simulink model "SpeedSimulationHW"  (R2013b)
settings: Solver=FixedStepDiscrete  SolverMode=SingleTasking  StartTime=0.0  StopTime=3000  FixedStep=0.1  RelTol=1e-3
undefined symbols (not defined in the file or in its folder): Sensor, spartan500lap_lib
libraries: xbsIndex_r4 x42, simulink x3
settings Model: Creator=laca  LastModifiedBy=laca

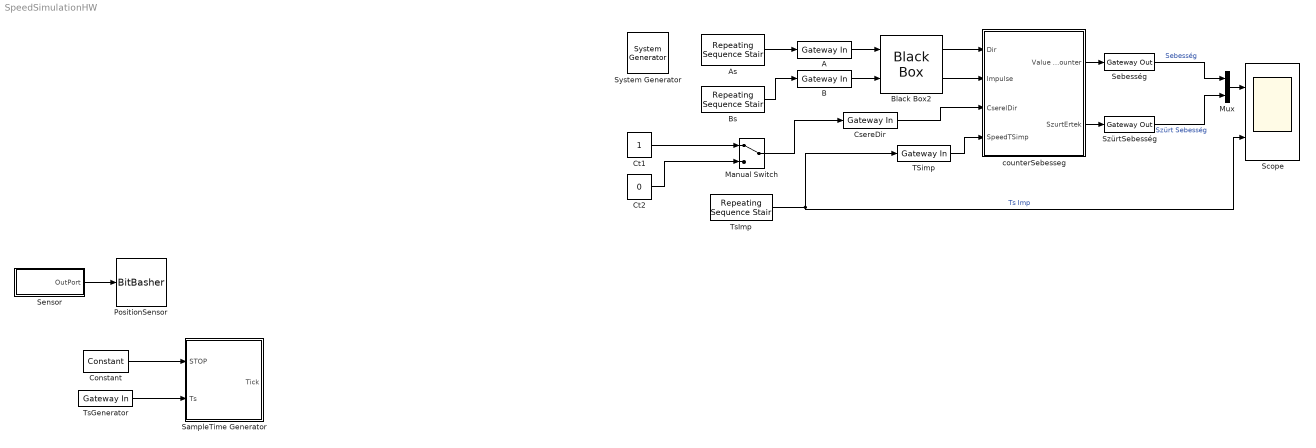
== system SpeedSimulationHW ==
  " System Generator" : xbsIndex_r4/ System Generator  Tag=genX  xilinxfamily=spartan3e  part=xc3s500e  speed=-4  package=pq208  synthesis_tool=XST  clock_wrapper=Clock Enables  directory=./netlist  proj_type=Project Navigator  Synth_file=XST Defaults  Impl_file=ISE Defaults  testbench=off  simulink_period=1  sysclk_period=20  dcm_input_clock_period=10  incr_netlist=off  trim_vbits=Everywhere in SubSystem  dbl_ovrd=According to Block Masks  core_generation=According to Block Masks  run_coregen=off  deprecated_control=off  eval_field=0  block_type=sysgen
  A : xbsIndex_r4/Gateway In  gui_display_data_type=Boolean  arith_type=Boolean  n_bits=16  bin_pt=14  preci_type=Single  exp_width=8  frac_width=24  quantization="Round  (unbiased: +/- Inf)"  overflow=Saturate  period=1  dbl_ovrd=off  timing_constraint=None  locs_specified=off  LOCs={}  UseAsADC=off  ADCChannel='1'  inherit_from_input=off  hdl_port=on  block_type=gatewayin
  As : simulink/Sources/Repeating Sequence Stair  OutValues="[ 0 0 1 1 1 1 1 0 0 0  0 0 1 1 1 1 1 0 0 0  0 0 1 1 1 1 1 0 0 0  0 0 1 1 1 1 1 0 0 0  0 0 1 1 1 1 1 0 0 0  0 0 1 1 1 1 1 0 0 0  0 0 1 1 1 1 1 0 0 0  0 0 1 1 1 1 1 0 0 0  0 0 1 1 1 1 1 0 0 0  0 0 1 1 1 1 1 0 0 0  0 0 1 1 1 1 1 0 0 0 0 0 1 1 1 1 1 0 0 0 0 0 1 1 1 1 1 0 0 0 0 0 1 1 1 1 1 0 0 0 1 1 1 1 1 0 0 0 0 0 1 1 1 1 1 0 0 0 0 0 1 1 1 1 1 0 0 0 0 0 1 1 1 1 1 0 0 0 0 0 0 0 0 1 1  0 0 0 0 0 0 0 0 1 1 0 0 0 0 0 0 0 0 1 1  0 0 0 0 0 0 0 0 1 1 0 0 0 0 0 0 0 0 0 0 0 0 0 0 0 0 0 0 0 0 0 0 0 0 0 0 0 0 0 0 0 0 0 0 0 0 0 0 0 0 0 0 0 0 0 0 1 1 0 0 0 0 0 0 0 0 1 1 0 0 0 0 0 0 0 0 1 1 0 0 0 0 ].'"  tsamp=1  OutMin=[]  OutMax=[]  OutDataTypeStr=double  OutputDataTypeScalingMode=double  OutDataType=fixdt(0,8)  ConRadixGroup=Best Precision: Vector-wise  OutScaling=2^-12
  B : xbsIndex_r4/Gateway In  gui_display_data_type=Boolean  arith_type=Boolean  n_bits=16  bin_pt=14  preci_type=Single  exp_width=8  frac_width=24  quantization="Round  (unbiased: +/- Inf)"  overflow=Saturate  period=1  dbl_ovrd=off  timing_constraint=None  locs_specified=off  LOCs={}  UseAsADC=off  ADCChannel='1'  inherit_from_input=off  hdl_port=on  block_type=gatewayin
  Black Box2 : xbsIndex_r4/Black Box  init_code=IncSensor_config  sim_method=ISE Simulator  verbose=off  block_type=blackbox2
  Bs : simulink/Sources/Repeating Sequence Stair  OutValues="[1 1 1 1 1 0 0 0 0 0 1 1 1 1 1 0 0 0 0 0 1 1 1 1 1 0 0 0 0 0 1 1 1 1 1 0 0 0 0 0 1 1 1 1 1 0 0 0 0 0 1 1 1 1 1 0 0 0 0 0 1 1 1 1 1 0 0 0 0 0 1 1 1 1 1 0 0 0 0 0 1 1 1 1 1 0 0 0 0 0 1 1 1 1 1 0 0 0 0 0 1 1 1 1 1 0 0 0 0 0 1 1 1 1 1 0 0 0 0 0 1 1 1 1 1 0 0 0 0 0 1 1 1 1 1 0 0 0 0 0 0 1 1 1 1 1 0 0 0 0 0 1 1 1 1 1 0 0 0 0 0 1 1 1 1 1 0 0 0 0 0 1 1 1 1 1 0 0 0  0 0 1 1 1 1 1 0 0 0  0 0 1 1 1 1 1 0 0 0  0 0 1 1 1 1 1 0 0 0  0 0 1 1 1 1 1 0 0 0  0 0 1 1 1 1 1 0 0 0  0 0 1 1 1 1 1 0 0 0 0 0 0 0 0 0 0 0 0 0 0 0 0 0 0 1 1 1 1 1 1 1 1 1 1 1 1 1 1 1 1 1 1 1 1 1 1 1 1 1 1 1 1 1 1].'"  tsamp=1  OutMin=[]  OutMax=[]  OutDataTypeStr=double  OutputDataTypeScalingMode=double  OutDataType=fixdt(0,8)  ConRadixGroup=Best Precision: Vector-wise  OutScaling=2^-12
  Constant : xbsIndex_r4/Constant  const=0  gui_display_data_type=Boolean  arith_type=Boolean  n_bits=16  bin_pt=14  preci_type=Single  exp_width=8  frac_width=24  explicit_period=off  period=1  equ=P=C  opselect=C  inp2=PCIN>>17  opr=+  inp1=P  carry=CIN  dbl_ovrd=off  block_type=constant
  CsereDir : xbsIndex_r4/Gateway In  gui_display_data_type=Boolean  arith_type=Boolean  n_bits=16  bin_pt=14  preci_type=Single  exp_width=8  frac_width=24  quantization="Round  (unbiased: +/- Inf)"  overflow=Saturate  period=1  dbl_ovrd=off  timing_constraint=None  locs_specified=off  LOCs={}  UseAsADC=off  ADCChannel='1'  inherit_from_input=off  hdl_port=on  block_type=gatewayin
  Ct1 : Constant
  Ct2 : Constant  Value=0
  Manual Switch : ManualSwitch
  Mux : Mux  Inputs=2
  PositionSensor : xbsIndex_r4/BitBasher  bitexpr=|  display_expr=off  sr_1=1  arith_type1=Unsigned  bin_pt1=0  sr_2=2  arith_type2=Unsigned  bin_pt2=0  sr_3=3  arith_type3=Unsigned  bin_pt3=0  sr_4=4  arith_type4=Unsigned  bin_pt4=0  dbl_ovrd=off  block_type=bitbasher
      | <!DOCTYPE HTML PUBLIC "-//W3C//DTD HTML 4.0//EN" "http://www.w3.org/TR/REC-html40/strict.dtd">
      | <html><head><meta name="qrichtext" content="1" /><style type="text/css">
      | p, li { white-space: pre-wrap; }
      | </style></head><body style=" font-family:'MS Shell Dlg 2'; font-size:8.25pt; font-weight:400; font-style:normal;">
      | <p style=" margin-top:12px; margin-bottom:12px; margin-left:0px; margin-right:0px; -qt-block-indent:0; text-indent:0px;"><span style=" font-family:'MS Shell Dlg'; font-size:8pt;">A={a[2]}<br />B={a[3]}</span></p></body></html>
  SampleTime Generator : Subsystem
  Scope : Scope  NumInputPorts=2
      settings: TickLabels=on  ShowLegends=on  YMin=225.15~-1  YMax=248.85~1
  Sebesség : xbsIndex_r4/Gateway Out  inherit_from_input=off  hdl_port=on  timing_constraint=None  locs_specified=off  LOCs={}  UseAsDAC=off  DACChannel='1'  block_type=gatewayout
  Sensor : Subsystem  AncestorBlock=spartan500lap_lib/Sensor  mask(Non-Memory-Mapped Input Port){signed=off, bpt=0, show_in=off, c=0}
      mask prompts: signed "Signed  (2's comp)"; bpt "Binary Point"; show_in "Provide Input Double"; c "Constant for Simulation"
      mask help:
      | Port Name: "Sensor"
      | Port Type: 5-bit Vector
      mask init:
      | [bg,fg] = xlcmap('IO',0);
      | iPos = get_param(gcb,'Position');
      | iWidth=iPos(3)-iPos(1);
      | iHeight=iPos(4)-iPos(2);
      | [logoX, logoY] = xlogo(iPos);
      | if (signed)
      |     set_param([gcb '/Sensor'],'arith_type','Signed  (2''s comp)');
      | else
      |     set_param([gcb '/Sensor'],'arith_type','Unsigned');
      | end
      | if (show_in)
      |     old = find_system(gcb, 'LookUnderMasks', 'all', 'Name', 'Constant');
      |     if (length(old) > 0)
      |         replace_block(gcb, 'Name', 'Constant', 'InPort', 'noprompt');
      |         set_param([gcb '/Constant'], 'Name', 'InPort');
      |     end
      |     portdir = 'input';
      |     portstr = 'dbl';
      | else
      |     old = find_system(gcb, 'LookUnderMasks', 'all', 'Name', 'InPort');
      |     if (length(old) > 0)
      |         replace_block(gcb, 'Name', 'InPort', 'Constant', 'noprompt');
      |         set_param([gcb '/InPort'], 'Name', 'Constant');
      |         set_param([gcb '/Constant'], 'Value', 'c');
      |     end
      |     portdir = 'output';
      |     portstr = '';
      | end
      settings: CopyFcn=set_param(gcb,'LinkStatus','inactive');
      mask Callback show_in:
      | mask_vis = get_param(gcb, 'MaskVisibilities');
      | if (strcmp(get_param(gcb, 'show_in'),'on'))
      |     mask_vis(4) = {'off'};
      | else
      |     mask_vis(4) = {'on'};
      | end
      | set_param(gcb, 'MaskVisibilities', mask_vis);
      mask Display:
      | patch([0 iWidth iWidth 0],[0 0 iHeight iHeight] , bg);
      | patch(logoX,logoY, fg);
      | plot([0 0 iWidth iWidth 0], [0 iHeight iHeight 0 0]);
      | port_label(portdir,1,portstr);
      | port_label('output',1,'Sensor');
      | text(2,5,'nmm');
  SzürtSebesség : xbsIndex_r4/Gateway Out  inherit_from_input=off  hdl_port=on  timing_constraint=None  locs_specified=off  LOCs={}  UseAsDAC=off  DACChannel='1'  block_type=gatewayout
  TSimp : xbsIndex_r4/Gateway In  gui_display_data_type=Boolean  arith_type=Boolean  n_bits=16  bin_pt=14  preci_type=Single  exp_width=8  frac_width=24  quantization="Round  (unbiased: +/- Inf)"  overflow=Saturate  period=1  dbl_ovrd=off  timing_constraint=None  locs_specified=off  LOCs={}  UseAsADC=off  ADCChannel='1'  inherit_from_input=off  hdl_port=on  block_type=gatewayin
  TsGenerator : xbsIndex_r4/Gateway In  gui_display_data_type=Fixed-point  arith_type="Signed  (2's comp)"  n_bits=16  bin_pt=14  preci_type=Single  exp_width=8  frac_width=24  quantization="Round  (unbiased: +/- Inf)"  overflow=Saturate  period=1  dbl_ovrd=off  timing_constraint=None  locs_specified=off  LOCs={}  UseAsADC=off  ADCChannel='1'  inherit_from_input=off  hdl_port=on  block_type=gatewayin
  TsImp : simulink/Sources/Repeating Sequence Stair  OutValues=[zeros(1,50) 1 ].'  tsamp=1  OutMin=[]  OutMax=[]  OutDataTypeStr=double  OutputDataTypeScalingMode=double  OutDataType=fixdt(0,8)  ConRadixGroup=Best Precision: Vector-wise  OutScaling=2^-12
  counterSebesseg : Subsystem
  wires:
  Sensor/1(OutPort) -> PositionSensor/1
  Constant/1 -> SampleTime Generator/1(STOP)
  TsGenerator/1 -> SampleTime Generator/2(Ts)
  Bs/1 -> B/1
  As/1 -> A/1
  A/1 -> Black Box2/1
  B/1 -> Black Box2/2
  Black Box2/1 -> counterSebesseg/1(Dir)
  Black Box2/2 -> counterSebesseg/2(Impulse)
  TSimp/1 -> counterSebesseg/4(SpeedTSimp)
  CsereDir/1 -> counterSebesseg/3(CserelDir)
  counterSebesseg/2(SzurtErtek) -> SzürtSebesség/1
  TsImp/1 -> TSimp/1, Scope/2  "Ts Imp"
  Ct1/1 -> Manual Switch/1
  Ct2/1 -> Manual Switch/2
  Sebesség/1 -> Mux/1  "Sebesség"
  SzürtSebesség/1 -> Mux/2  "Szürt Sebesség"
  Mux/1 -> Scope/1
  Manual Switch/1 -> CsereDir/1
  counterSebesseg/1(Value Counter) -> Sebesség/1

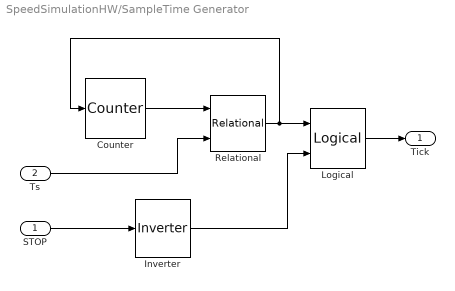
== system SpeedSimulationHW/SampleTime Generator ==
  STOP : Inport
  Ts : Inport  Port=2
  Counter : xbsIndex_r4/Counter  cnt_type=Free Running  cnt_to=Inf  operation=Up  start_count=0  cnt_by_val=1  arith_type=Unsigned  n_bits=32  bin_pt=0  load_pin=off  rst=on  en=off  explicit_period=on  period=1  dbl_ovrd=off  use_behavioral_HDL=off  implementation=Fabric  block_type=counter
  Inverter : xbsIndex_r4/Inverter  en=off  latency=0  dbl_ovrd=off  block_type=inv
  Logical : xbsIndex_r4/Logical  logical_function=AND  inputs=2  en=off  latency=0  precision=Full  arith_type=Unsigned  n_bits=16  bin_pt=0  align_bp=on  dbl_ovrd=off  block_type=logical
  Relational : xbsIndex_r4/Relational  mode=a=b  en=off  latency=0  dbl_ovrd=off  block_type=relational
  Tick : Outport
  wires:
  Ts/1 -> Relational/2
  Counter/1 -> Relational/1
  Relational/1 -> Logical/1, Counter/1
  Logical/1 -> Tick/1
  STOP/1 -> Inverter/1
  Inverter/1 -> Logical/2

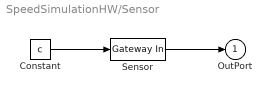
== system SpeedSimulationHW/Sensor ==
  Constant : Constant  Value=c
  Sensor : xbsIndex_r4/Gateway In  gui_display_data_type=Fixed-point  arith_type=Unsigned  n_bits=5  bin_pt=max(0,min(bpt,5))  preci_type=Single  exp_width=8  frac_width=24  quantization="Round  (unbiased: +/- Inf)"  overflow=Saturate  period=1  dbl_ovrd=off  timing_constraint=None  locs_specified=on  LOCs={'P112','P113','P115','P116','P119'}  UseAsADC=off  ADCChannel='1'  inherit_from_input=off  hdl_port=on  block_type=gatewayin
      settings: sginterface={'Xilinx'=>{'jtaghwcosim'=>{'non_memory_mapped_port'=>'Sensor'}}}
  OutPort : Outport
  wires:
  Sensor/1 -> OutPort/1
  Constant/1 -> Sensor/1

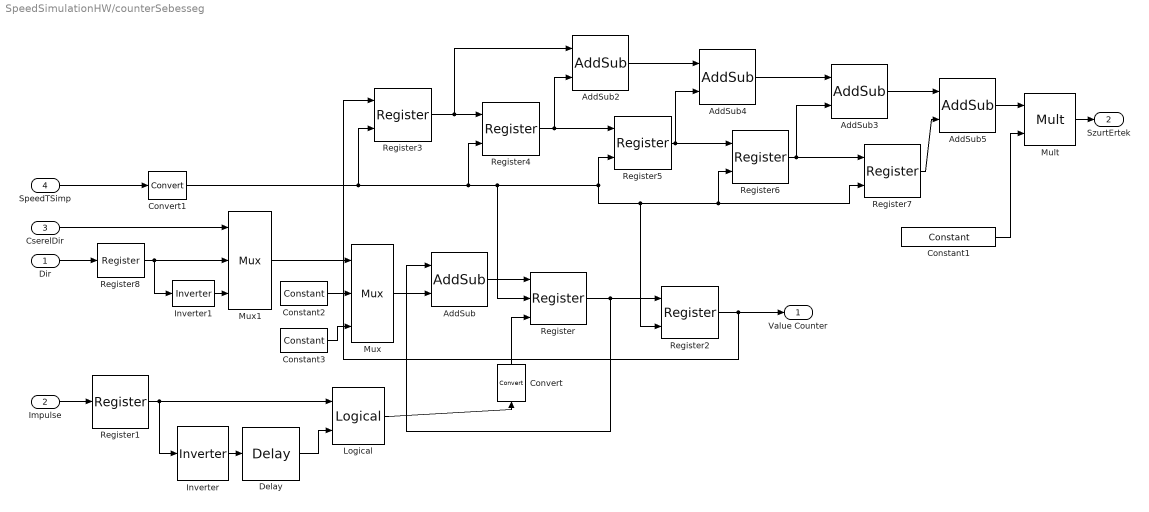
== system SpeedSimulationHW/counterSebesseg ==
  Dir : Inport
  Impulse : Inport  Port=2
  CserelDir : Inport  Port=3
  SpeedTSimp : Inport  Port=4
  AddSub{,2..5} (5 alike) : xbsIndex_r4/AddSub  mode=Addition  use_carryin=off  use_carryout=off  en=off  latency=0  precision=User Defined  arith_type="Signed  (2's comp)"  n_bits=16  bin_pt=0  quantization=Truncate  overflow=Saturate  dbl_ovrd=off  use_behavioral_HDL=off  hw_selection=Fabric  pipelined=off  block_type=addsub
  Constant1 : xbsIndex_r4/Constant  const=1/5  gui_display_data_type=Fixed-point  arith_type=Signed (2's comp)  n_bits=16  bin_pt=14  preci_type=Single  exp_width=8  frac_width=24  explicit_period=off  period=1  equ=P=C  opselect=C  inp2=PCIN>>17  opr=+  inp1=P  carry=CIN  dbl_ovrd=off  block_type=constant
  Constant2 : xbsIndex_r4/Constant  const=-1  gui_display_data_type=Fixed-point  arith_type=Signed (2's comp)  n_bits=16  bin_pt=0  preci_type=Single  exp_width=8  frac_width=24  explicit_period=off  period=1  equ=P=C  opselect=C  inp2=PCIN>>17  opr=+  inp1=P  carry=CIN  dbl_ovrd=off  block_type=constant
  Constant3 : xbsIndex_r4/Constant  const=1  gui_display_data_type=Fixed-point  arith_type=Signed (2's comp)  n_bits=16  bin_pt=0  preci_type=Single  exp_width=8  frac_width=24  explicit_period=off  period=1  equ=P=C  opselect=C  inp2=PCIN>>17  opr=+  inp1=P  carry=CIN  dbl_ovrd=off  block_type=constant
  Convert : xbsIndex_r4/Convert  gui_display_data_type=Boolean  arith_type=Boolean  n_bits=16  bin_pt=14  float_type=Single  exp_bits=8  fraction_bits=24  quantization=Truncate  overflow=Wrap  en=off  latency=0  dbl_ovrd=off  pipeline=off  block_type=convert
  Convert1 : xbsIndex_r4/Convert  gui_display_data_type=Boolean  arith_type=Boolean  n_bits=16  bin_pt=14  float_type=Single  exp_bits=8  fraction_bits=24  quantization=Truncate  overflow=Wrap  en=off  latency=0  dbl_ovrd=off  pipeline=off  block_type=convert
  Delay : xbsIndex_r4/Delay  rst=off  infoeditControl=Selection of Reset will increase slice count due to use of real FFs and instead of SRLs  en=off  latency=1  dbl_ovrd=off  reg_retiming=off  block_type=delay
  Inverter : xbsIndex_r4/Inverter  en=off  latency=0  dbl_ovrd=off  block_type=inv
  Inverter1 : xbsIndex_r4/Inverter  en=off  latency=0  dbl_ovrd=off  block_type=inv
  Logical : xbsIndex_r4/Logical  logical_function=AND  inputs=2  en=off  latency=0  precision=Full  arith_type=Unsigned  n_bits=16  bin_pt=0  align_bp=on  dbl_ovrd=off  block_type=logical
  Mult : xbsIndex_r4/Mult  precision=User Defined  arith_type="Signed  (2's comp)"  n_bits=16  bin_pt=0  quantization=Truncate  overflow=Saturate  en=off  latency=1  dbl_ovrd=off  use_behavioral_HDL=off  opt=Speed  use_embedded=on  optimum_pipeline=off  pipeline=on  use_rpm=on  placement_style=Triangular  block_type=mult
  Mux : xbsIndex_r4/Mux  inputs=2  en=off  latency=0  precision=User Defined  arith_type="Signed  (2's comp)"  n_bits=16  bin_pt=0  quantization=Truncate  overflow=Saturate  dbl_ovrd=off  block_type=mux
  Mux1 : xbsIndex_r4/Mux  inputs=2  en=off  latency=0  precision=User Defined  arith_type=Unsigned  n_bits=1  bin_pt=0  quantization=Truncate  overflow=Saturate  dbl_ovrd=off  block_type=mux
  Register : xbsIndex_r4/Register  init=0  rst=on  en=on  dbl_ovrd=off  block_type=register
  Register1 : xbsIndex_r4/Register  init=0  rst=off  en=off  dbl_ovrd=off  block_type=register
  Register{2..7} (6 alike) : xbsIndex_r4/Register  init=0  rst=off  en=on  dbl_ovrd=off  block_type=register
  Register8 : xbsIndex_r4/Register  init=0  rst=off  en=off  dbl_ovrd=off  block_type=register
  Value Counter : Outport
  SzurtErtek : Outport  Port=2
  wires:
  Register2/1 -> Register3/1, Value Counter/1
  Register3/1 -> Register4/1, AddSub2/1
  Register4/1 -> Register5/1, AddSub2/2
  Register5/1 -> AddSub4/2, Register6/1
  AddSub2/1 -> AddSub4/1
  Constant1/1 -> Mult/2
  Mult/1 -> SzurtErtek/1
  Register6/1 -> Register7/1, AddSub3/2
  AddSub4/1 -> AddSub3/1
  AddSub3/1 -> AddSub5/1
  Register7/1 -> AddSub5/2
  AddSub5/1 -> Mult/1
  Constant3/1 -> Mux/3
  Dir/1 -> Register8/1
  Inverter/1 -> Delay/1
  Delay/1 -> Logical/2
  Logical/1 -> Convert/1
  Impulse/1 -> Register1/1
  Register/1 -> AddSub/1, Register2/1
  Convert/1 -> Register/3
  Convert1/1 -> Register2/2, Register6/2, Register7/2, Register5/2, Register/2, Register4/2, Register3/2
  Register1/1 -> Logical/1, Inverter/1
  AddSub/1 -> Register/1
  Mux/1 -> AddSub/2
  Constant2/1 -> Mux/2
  Register8/1 -> Inverter1/1, Mux1/2
  Mux1/1 -> Mux/1
  CserelDir/1 -> Mux1/1
  Inverter1/1 -> Mux1/3
  SpeedTSimp/1 -> Convert1/1
